simulink model "PID_controlledPosiotioning"  (R2015a)
settings: Solver=ode45  StartTime=0.0  StopTime=inf  RelTol=1e-3
libraries: robotlib x6
settings Model: Creator=root  LastModifiedBy=root

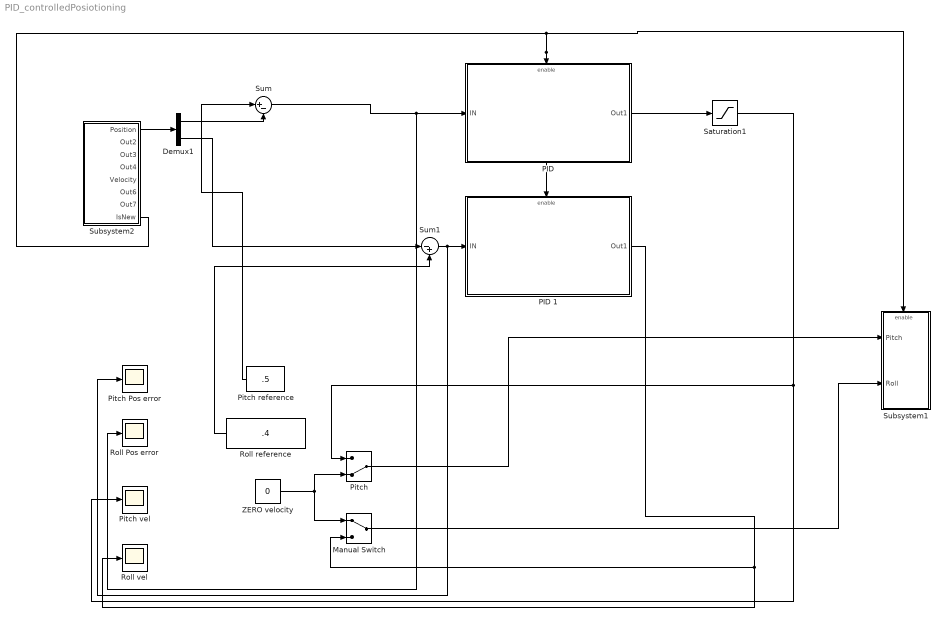
== system PID_controlledPosiotioning ==
  Demux1 : Demux  Outputs=2
  Manual Switch : ManualSwitch
  "PID " : Subsystem
  PID 1 : Subsystem
  Pitch : ManualSwitch  CurrentSetting=0
  "Pitch Pos error " : Scope
      settings: TimeRange=10  YMin=-40  YMax=30  SaveName=commandVelocity1
  Pitch reference : Constant  Value=.5
  Pitch vel : Scope
      settings: TimeRange=10  YMin=-40  YMax=30  SaveName=commandVelocity
  Roll Pos error : Scope
      settings: TimeRange=10  YMin=-0.0031  YMax=-0.0015  SaveName=commandVelocity3
  Roll reference : Constant  Value=.4
  Roll vel : Scope
      settings: TimeRange=10  YMin=-1  YMax=1.4  SaveName=commandVelocity2
  Saturation1 : Saturate  UpperLimit=3  LowerLimit=-3
  Subsystem1 : Subsystem
  Subsystem2 : Subsystem
  Sum : Sum  Inputs=|+-
  Sum1 : Sum  Inputs=|-+
  "ZERO velocity " : Constant  Value=0
  wires:
  "PID "/1(Out1) -> Saturation1/1
  Subsystem2/1("Position ") -> Demux1/1
  Pitch reference/1 -> Sum/1
  Sum/1 -> Roll Pos error/1, "PID "/1(IN)
  Subsystem2/8("IsNew ") -> PID 1/Enable, "PID "/Enable, Subsystem1/Enable
  Saturation1/1 -> Pitch/1, Pitch vel/1
  Roll reference/1 -> Sum1/2
  Demux1/2 -> Sum1/1
  Sum1/1 -> "Pitch Pos error "/1, PID 1/1(IN)
  PID 1/1(Out1) -> Roll vel/1, Manual Switch/2
  Pitch/1 -> Subsystem1/1(Pitch)
  Manual Switch/1 -> Subsystem1/2(Roll)
  "ZERO velocity "/1 -> Manual Switch/1, Pitch/2
  Demux1/1 -> Sum/2

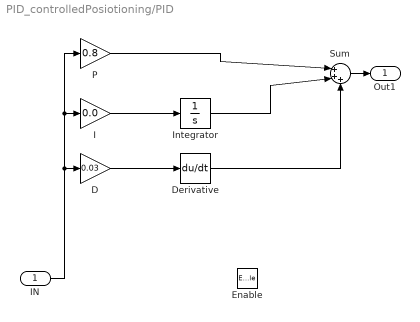
== system PID_controlledPosiotioning/PID  ==
  IN : Inport
  Enable : EnablePort
  D : Gain  Gain=0.03
  Derivative : Derivative
  I : Gain  Gain=0.0
  Integrator : Integrator
  "P " : Gain  Gain=0.8
  Sum : Sum  Inputs=|+++
  Out1 : Outport
  wires:
  D/1 -> Derivative/1
  "P "/1 -> Sum/1
  IN/1 -> D/1, I/1, "P "/1
  I/1 -> Integrator/1
  Sum/1 -> Out1/1
  Integrator/1 -> Sum/2
  Derivative/1 -> Sum/3

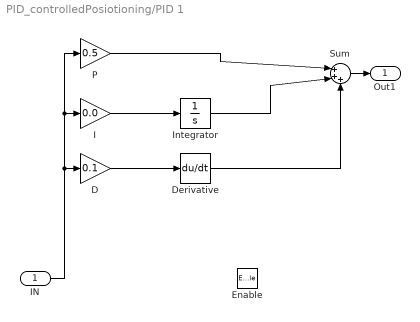
== system PID_controlledPosiotioning/PID 1 ==
  IN : Inport
  Enable : EnablePort
  D : Gain  Gain=0.1
  Derivative : Derivative
  I : Gain  Gain=0.0
  Integrator : Integrator
  "P " : Gain  Gain=0.5
  Sum : Sum  Inputs=|+++
  Out1 : Outport
  wires:
  Derivative/1 -> Sum/3
  Integrator/1 -> Sum/2
  Sum/1 -> Out1/1
  I/1 -> Integrator/1
  IN/1 -> "P "/1, I/1, D/1
  "P "/1 -> Sum/1
  D/1 -> Derivative/1

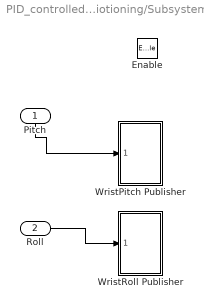
== system PID_controlledPosiotioning/Subsystem1 ==
  Pitch : Inport
  Roll : Inport  Port=2
  Enable : EnablePort
  WristPitch Publisher : Subsystem
  "WristRoll Publisher " : Subsystem
  wires:
  Pitch/1 -> WristPitch Publisher/1(velocity)
  Roll/1 -> "WristRoll Publisher "/1(velocity)

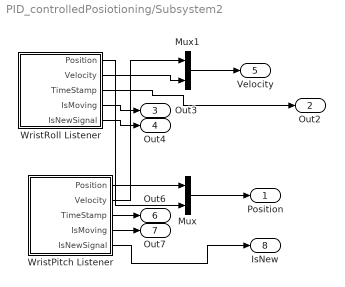
== system PID_controlledPosiotioning/Subsystem2 ==
  Mux : Mux  Inputs=2
  Mux1 : Mux  Inputs=2
  WristPitch Listener : Subsystem
  WristRoll Listener : Subsystem
  "Position " : Outport
  Out2 : Outport  Port=2
  Out3 : Outport  Port=3
  Out4 : Outport  Port=4
  Velocity : Outport  Port=5
  Out6 : Outport  Port=6
  Out7 : Outport  Port=7
  "IsNew " : Outport  Port=8
  wires:
  WristPitch Listener/3(TimeStamp) -> Out6/1
  Mux/1 -> "Position "/1
  WristPitch Listener/5(IsNewSignal) -> "IsNew "/1
  WristRoll Listener/5(IsNewSignal) -> Out4/1
  WristRoll Listener/3(TimeStamp) -> Out2/1
  Mux1/1 -> Velocity/1
  WristRoll Listener/4("IsMoving ") -> Out3/1
  WristPitch Listener/4("IsMoving ") -> Out7/1
  WristPitch Listener/1(Position) -> Mux/1
  WristPitch Listener/2(Velocity) -> Mux1/1
  WristRoll Listener/1(Position) -> Mux/2
  WristRoll Listener/2(Velocity) -> Mux1/2

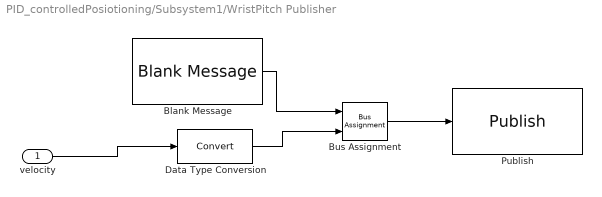
== system PID_controlledPosiotioning/Subsystem1/WristPitch Publisher ==
  velocity : Inport
  Blank Message : robotlib/Blank Message  SourceLibraryInfo=This block requires Robotics System Toolbox  messageType=std_msgs/Float64  SampleTime=inf
  Bus Assignment : BusAssignment  AssignedSignals=Data
  Data Type Conversion : DataTypeConversion
  Publish : robotlib/Publish  SourceLibraryInfo=This block requires Robotics System Toolbox  topicSource=Specify your own  topic=/wrist_pitch_speed_controller/command  messageType=std_msgs/Float64  messageQueueLength=1
  wires:
  velocity/1 -> Data Type Conversion/1
  Blank Message/1 -> Bus Assignment/1
  Bus Assignment/1 -> Publish/1
  Data Type Conversion/1 -> Bus Assignment/2

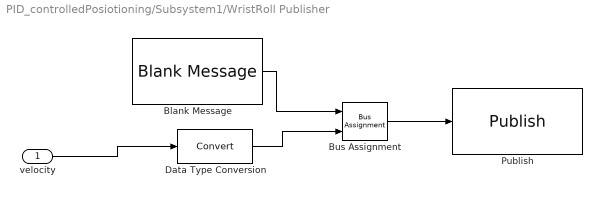
== system PID_controlledPosiotioning/Subsystem1/WristRoll Publisher  ==
  velocity : Inport
  Blank Message : robotlib/Blank Message  SourceLibraryInfo=This block requires Robotics System Toolbox  messageType=std_msgs/Float64  SampleTime=inf
  Bus Assignment : BusAssignment  AssignedSignals=Data
  Data Type Conversion : DataTypeConversion
  Publish : robotlib/Publish  SourceLibraryInfo=This block requires Robotics System Toolbox  topicSource=Specify your own  topic=/wrist_roll_speed_controller/command  messageType=std_msgs/Float64  messageQueueLength=1
  wires:
  Data Type Conversion/1 -> Bus Assignment/2
  Bus Assignment/1 -> Publish/1
  Blank Message/1 -> Bus Assignment/1
  velocity/1 -> Data Type Conversion/1

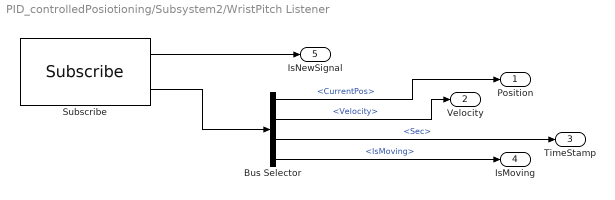
== system PID_controlledPosiotioning/Subsystem2/WristPitch Listener ==
  Bus Selector : BusSelector  OutputSignals=CurrentPos,Velocity,Header.Stamp.Sec,IsMoving
  Subscribe : robotlib/Subscribe  SourceLibraryInfo=This block requires Robotics System Toolbox  topicSource=Select from ROS network  topic=/wrist_pitch_speed_controller/state  messageType=dynamixel_msgs/JointState  sampleTime=-1  messageQueueLength=1
  Position : Outport
  Velocity : Outport  Port=2
  TimeStamp : Outport  Port=3
  "IsMoving " : Outport  Port=4
  IsNewSignal : Outport  Port=5
  wires:
  Bus Selector/4 -> "IsMoving "/1  "<IsMoving>"
  Subscribe/2 -> Bus Selector/1
  Bus Selector/1 -> Position/1  "<CurrentPos>"
  Bus Selector/2 -> Velocity/1  "<Velocity>"
  Bus Selector/3 -> TimeStamp/1  "<Sec>"
  Subscribe/1 -> IsNewSignal/1

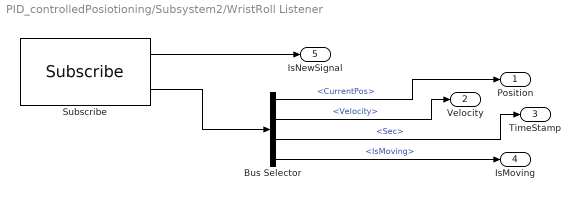
== system PID_controlledPosiotioning/Subsystem2/WristRoll Listener ==
  Bus Selector : BusSelector  OutputSignals=CurrentPos,Velocity,Header.Stamp.Sec,IsMoving
  Subscribe : robotlib/Subscribe  SourceLibraryInfo=This block requires Robotics System Toolbox  topicSource=Select from ROS network  topic=/wrist_roll_speed_controller/state  messageType=dynamixel_msgs/JointState  sampleTime=-1  messageQueueLength=1
  Position : Outport
  Velocity : Outport  Port=2
  TimeStamp : Outport  Port=3
  "IsMoving " : Outport  Port=4
  IsNewSignal : Outport  Port=5
  wires:
  Subscribe/1 -> IsNewSignal/1
  Bus Selector/3 -> TimeStamp/1  "<Sec>"
  Bus Selector/2 -> Velocity/1  "<Velocity>"
  Bus Selector/1 -> Position/1  "<CurrentPos>"
  Subscribe/2 -> Bus Selector/1
  Bus Selector/4 -> "IsMoving "/1  "<IsMoving>"
